simulink model "unstable_sim"  (R2021a)
settings: Solver=VariableStepAuto  StartTime=0.0  StopTime=10  RelTol=1e-3
values from neighbouring files (symbols this model uses):
  alpha_0 = 0.9*pi    (= 2.82743338823)    [unstable_simulator.m]
  K = lqr(A,B,Q,R)    [unstable_init.m]
  Q = diag([1 1 1 1])    [unstable_init.m]
  R = 1    [unstable_init.m]
undefined symbols (not defined in the file or in its folder): bp, br, g, Jp, Jr, l, mp, r
settings Model: Creator=willi  LastModifiedBy=magd4814

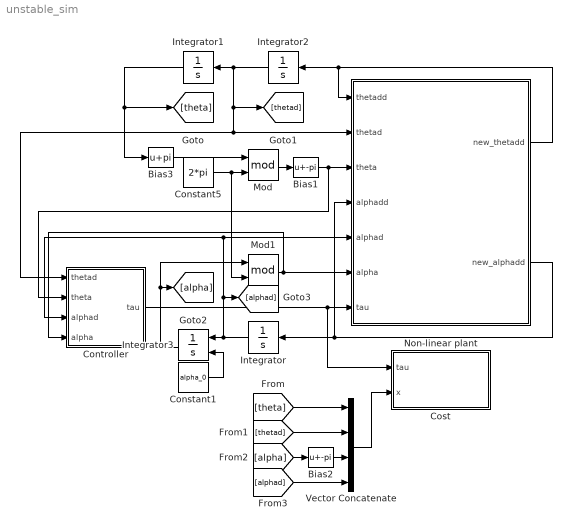
== system unstable_sim ==
  Bias1 : Bias  Bias=-pi
  Bias2 : Bias  Bias=-pi
  Bias3 : Bias  Bias=pi
  Constant1 : Constant  Value=alpha_0
  Constant5 : Constant  Value=2*pi
  Controller : Subsystem
  Cost : Subsystem
  Integrator : Integrator
  Integrator1 : Integrator
  Integrator2 : Integrator
  Integrator3 : Integrator  InitialConditionSource=external
  Mod : Math  Operator=mod  SaturateOnIntegerOverflow=on
  Mod1 : Math  Operator=mod  SaturateOnIntegerOverflow=on
  Non-linear plant : Subsystem
  Vector Concatenate : Concatenate  NumInputs=4
  wires:
  Non-linear plant/1(new_thetadd) -> Integrator2/1, Non-linear plant/1(thetadd)
  Non-linear plant/2(new_alphadd) -> Integrator/1, Non-linear plant/4(alphadd)
  Constant1/1 -> Integrator3/2
  Constant5/1 -> Mod1/2, Mod/2
  Mod/1 -> Bias1/1
  Integrator1/1 -> [theta], Bias3/1
  Bias3/1 -> Mod/1
  Integrator3/1 -> [alpha], Mod1/1
  Bias1/1 -> Controller/2(theta), Non-linear plant/3(theta)
  Integrator/1 -> [alphad], Non-linear plant/5(alphad), Controller/3(alphad), Integrator3/1
  Mod1/1 -> Non-linear plant/6(alpha), Controller/4(alpha)
  Integrator2/1 -> Controller/1(thetad), Non-linear plant/2(thetad), [thetad], Integrator1/1
  [thetad] -> Vector Concatenate/2
  Vector Concatenate/1 -> Cost/2(x)
  [alphad] -> Vector Concatenate/4
  Controller/1(tau) -> Cost/1(tau), Non-linear plant/7(tau)
  [theta] -> Vector Concatenate/1
  [alpha] -> Bias2/1
  Bias2/1 -> Vector Concatenate/3

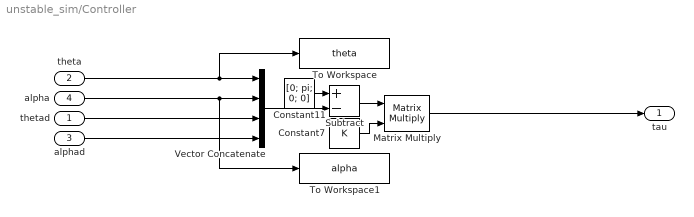
== system unstable_sim/Controller ==
  thetad : Inport
  theta : Inport  Port=2
  alphad : Inport  Port=3
  alpha : Inport  Port=4
  Constant11 : Constant  Value=[0; pi; 0; 0]
  Constant7 : Constant  Value=K
  Matrix Multiply : Product  Multiplication=Matrix(*)
  Subtract : Sum  Inputs=+-
  To Workspace : ToWorkspace  VariableName=theta  SaveFormat=Timeseries  SampleTime=-1
  To Workspace1 : ToWorkspace  VariableName=alpha  SaveFormat=Timeseries  SampleTime=-1
  Vector Concatenate : Concatenate  NumInputs=4
  tau : Outport
  wires:
  thetad/1 -> Vector Concatenate/3
  alpha/1 -> To Workspace1/1, Vector Concatenate/2
  Constant11/1 -> Subtract/1
  Subtract/1 -> Matrix Multiply/1
  Constant7/1 -> Matrix Multiply/2
  theta/1 -> To Workspace/1, Vector Concatenate/1
  Vector Concatenate/1 -> Subtract/2
  Matrix Multiply/1 -> tau/1
  alphad/1 -> Vector Concatenate/4

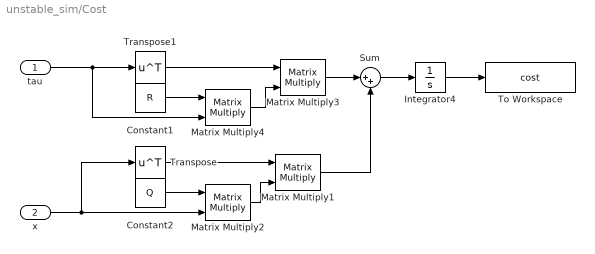
== system unstable_sim/Cost ==
  tau : Inport
  x : Inport  Port=2
  Constant1 : Constant  Value=R
  Constant2 : Constant  Value=Q
  Integrator4 : Integrator
  Matrix Multiply{1..4} (4 alike) : Product  Multiplication=Matrix(*)
  Sum : Sum  Inputs=|++
  To Workspace : ToWorkspace  VariableName=cost  SaveFormat=Timeseries  SampleTime=-1
  Transpose : Math  Operator=transpose  SaturateOnIntegerOverflow=on
  Transpose1 : Math  Operator=transpose  SaturateOnIntegerOverflow=on
  wires:
  Transpose/1 -> Matrix Multiply1/1
  Matrix Multiply2/1 -> Matrix Multiply1/2
  Integrator4/1 -> To Workspace/1
  x/1 -> Matrix Multiply2/2, Transpose/1
  Constant2/1 -> Matrix Multiply2/1
  Matrix Multiply1/1 -> Sum/2
  Sum/1 -> Integrator4/1
  Matrix Multiply3/1 -> Sum/1
  Constant1/1 -> Matrix Multiply4/1
  Transpose1/1 -> Matrix Multiply3/1
  Matrix Multiply4/1 -> Matrix Multiply3/2
  tau/1 -> Matrix Multiply4/2, Transpose1/1

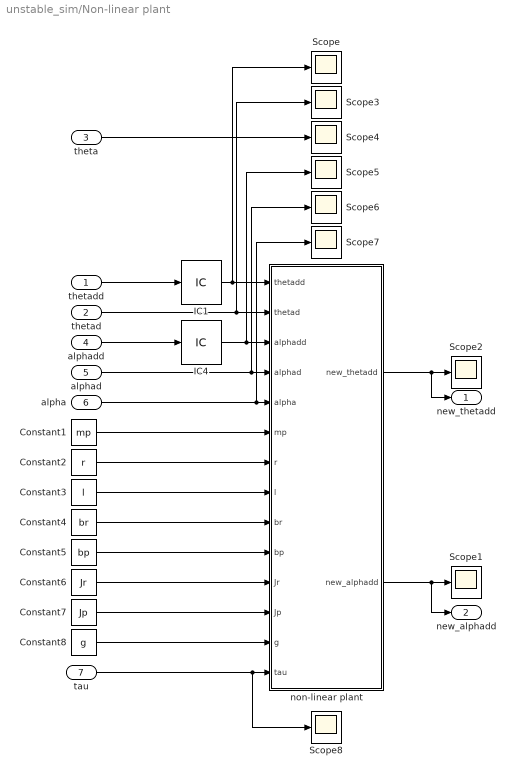
== system unstable_sim/Non-linear plant ==
  thetadd : Inport
  thetad : Inport  Port=2
  theta : Inport  Port=3
  alphadd : Inport  Port=4
  alphad : Inport  Port=5
  alpha : Inport  Port=6
  tau : Inport  Port=7
  Constant1 : Constant  Value=mp
  Constant2 : Constant  Value=r
  Constant3 : Constant  Value=l
  Constant4 : Constant  Value=br
  Constant5 : Constant  Value=bp
  Constant6 : Constant  Value=Jr
  Constant7 : Constant  Value=Jp
  Constant8 : Constant  Value=g
  IC1 : InitialCondition  Value=0
  IC4 : InitialCondition  Value=0
  Scope{,1..8} (9 alike) : Scope
  non-linear plant : MATLAB Function  TreatAsAtomicUnit=on
  new_thetadd : Outport
  new_alphadd : Outport  Port=2
  wires:
  Constant3/1 -> non-linear plant/8(l)
  Constant2/1 -> non-linear plant/7(r)
  alphad/1 -> Scope6/1, non-linear plant/4(alphad)
  non-linear plant/1(new_thetadd) -> new_thetadd/1, Scope2/1
  alpha/1 -> Scope7/1, non-linear plant/5(alpha)
  Constant1/1 -> non-linear plant/6(mp)
  Constant7/1 -> non-linear plant/12(Jp)
  non-linear plant/2(new_alphadd) -> new_alphadd/1, Scope1/1
  Constant5/1 -> non-linear plant/10(bp)
  theta/1 -> Scope4/1
  Constant4/1 -> non-linear plant/9(br)
  Constant8/1 -> non-linear plant/13(g)
  Constant6/1 -> non-linear plant/11(Jr)
  alphadd/1 -> IC4/1
  IC1/1 -> Scope/1, non-linear plant/1(thetadd)
  IC4/1 -> Scope5/1, non-linear plant/3(alphadd)
  tau/1 -> Scope8/1, non-linear plant/14(tau)
  thetad/1 -> Scope3/1, non-linear plant/2(thetad)
  thetadd/1 -> IC1/1

== matlab function unstable_sim/Non-linear plant/non-linear plant ==
  data: thetadd input; thetad input; new_thetadd output; alphadd input; alphad input; alpha input; mp input; r input; l input; br input; bp input; Jr input; Jp input; g input; tau input; new_alphadd output
function [new_thetadd, new_alphadd]= fcn(thetadd, thetad, alphadd, alphad, alpha, mp, r, l, br, bp, Jr, Jp, g, tau)

new_alphadd = (-bp*alphad - mp*g*l*sin(alpha) + Jp*(thetad^2)*sin(alpha)*cos(alpha) - mp*l*r*thetadd*cos(alpha)) / Jp;
new_thetadd = (tau - br*thetad + mp*l*r*(alphad^2)*sin(alpha) - 2*Jp*alphad*thetad*sin(alpha)*cos(alpha) - mp*l*r*alphadd*cos(alpha)) / (Jr+Jp*(sin(alpha)^2));
